simulink model "Assignment3"  (R2014a)
settings: Solver=FixedStepDiscrete  StartTime=0.0  StopTime=2000  FixedStep=1  RelTol=1e-3
libraries: simulink x4, hdlsllib x4
settings Model: Creator=vu.du  LastModifiedBy=vu.du

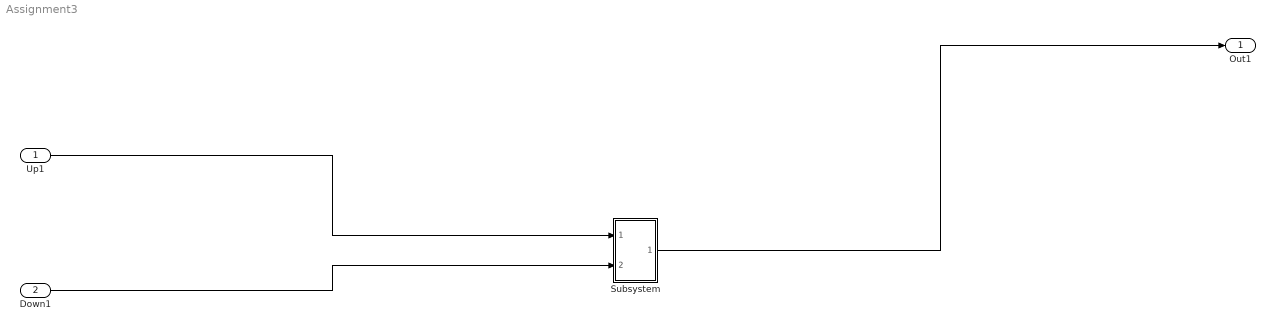
== system Assignment3 ==
  Up1 : Inport
  Down1 : Inport  Port=2
  Subsystem : Subsystem  TreatAsAtomicUnit=on
  Out1 : Outport
  wires:
  Up1/1 -> Subsystem/1(Up1)
  Down1/1 -> Subsystem/2(Down1)
  Subsystem/1(Out1) -> Out1/1

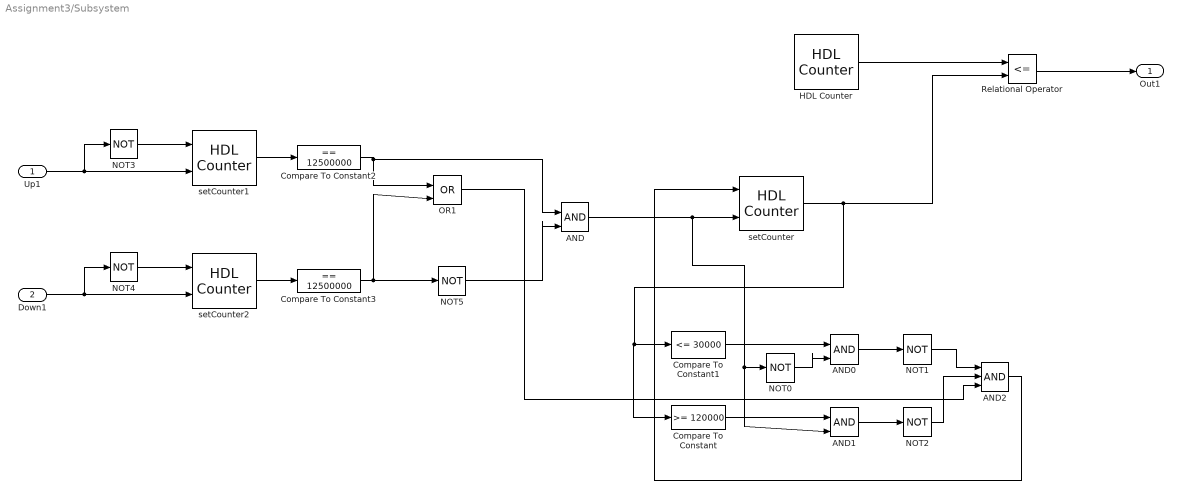
== system Assignment3/Subsystem ==
  Up1 : Inport
  Down1 : Inport  Port=2
  AND : Logic  IconShape=distinctive  AllPortsSameDT=off  OutDataTypeStr=boolean
  AND0 : Logic  IconShape=distinctive  AllPortsSameDT=off  OutDataTypeStr=boolean
  AND1 : Logic  IconShape=distinctive  AllPortsSameDT=off  OutDataTypeStr=boolean
  AND2 : Logic  Inputs=3  IconShape=distinctive  AllPortsSameDT=off  OutDataTypeStr=boolean
  Compare To Constant : simulink/Logic and Bit Operations/Compare To Constant  relop=>=  const=120000  OutDataTypeStr=boolean
  Compare To Constant1 : simulink/Logic and Bit Operations/Compare To Constant  relop=<=  const=30000  OutDataTypeStr=boolean
  Compare To Constant2 : simulink/Logic and Bit Operations/Compare To Constant  relop===  const=12500000  OutDataTypeStr=boolean
  Compare To Constant3 : simulink/Logic and Bit Operations/Compare To Constant  relop===  const=12500000  OutDataTypeStr=boolean
  HDL Counter : hdlsllib/HDL Operations/HDL Counter  CountType=Count limited  CountInit=0  CountStep=1  CountMax=1000000  CountFromType=Initial value  CountFrom=0  CountResetPort=off  CountLoadPort=off  CountEnbPort=off  CountDirPort=off  CountDataType=Unsigned  CountWordLen=32  CountFracLen=0  CountSampTime=1
  NOT{0..5} (6 alike) : Logic  Operator=NOT  IconShape=distinctive  AllPortsSameDT=off  OutDataTypeStr=boolean
  OR1 : Logic  Operator=OR  IconShape=distinctive  AllPortsSameDT=off  OutDataTypeStr=boolean
  Relational Operator : RelationalOperator  Operator=<=  OutDataTypeStr=boolean
  setCounter : hdlsllib/HDL Operations/HDL Counter  CountType=Count limited  CountInit=75000  CountStep=6000  CountMax=120000  CountFromType=Specify  CountFrom=30000  CountResetPort=off  CountLoadPort=off  CountEnbPort=on  CountDirPort=on  CountDataType=Unsigned  CountWordLen=32  CountFracLen=0  CountSampTime=1
  setCounter1 : hdlsllib/HDL Operations/HDL Counter  CountType=Count limited  CountInit=0  CountStep=1  CountMax=50000000  CountFromType=Initial value  CountFrom=0  CountResetPort=on  CountLoadPort=off  CountEnbPort=on  CountDirPort=off  CountDataType=Unsigned  CountWordLen=32  CountFracLen=0  CountSampTime=1
  setCounter2 : hdlsllib/HDL Operations/HDL Counter  CountType=Count limited  CountInit=0  CountStep=1  CountMax=50000000  CountFromType=Initial value  CountFrom=0  CountResetPort=on  CountLoadPort=off  CountEnbPort=on  CountDirPort=off  CountDataType=Unsigned  CountWordLen=32  CountFracLen=0  CountSampTime=1
  Out1 : Outport
  wires:
  Up1/1 -> setCounter1/2, NOT3/1
  Compare To Constant1/1 -> AND0/1
  NOT0/1 -> AND0/2
  AND2/1 -> setCounter/1
  Compare To Constant/1 -> AND1/1
  NOT1/1 -> AND2/1
  AND0/1 -> NOT1/1
  AND1/1 -> NOT2/1
  AND/1 -> AND1/2, NOT0/1, setCounter/2
  NOT2/1 -> AND2/2
  Relational Operator/1 -> Out1/1
  setCounter/1 -> Compare To Constant/1, Compare To Constant1/1, Relational Operator/2
  HDL Counter/1 -> Relational Operator/1
  Down1/1 -> setCounter2/2, NOT4/1
  NOT4/1 -> setCounter2/1
  setCounter2/1 -> Compare To Constant3/1
  Compare To Constant3/1 -> NOT5/1, OR1/2
  OR1/1 -> AND2/3
  setCounter1/1 -> Compare To Constant2/1
  Compare To Constant2/1 -> AND/1, OR1/1
  NOT3/1 -> setCounter1/1
  NOT5/1 -> AND/2
